simulink model "LQR_Controller_Quadrotor"  (R2019b)
settings: Solver=VariableStepAuto  StartTime=0.0  StopTime=10.0  RelTol=1e-3
values from neighbouring files (symbols this model uses):
  A = [ 0 0 0 1 0 0 0 0 0 0 0 0 ... (first row only)    [LQR control.m]
  B = [ 0 0 0 0 ... (first row only)    [LQR control.m]
  b = 6.66e-5    (= 6.66e-05)    [LQR control.m]    (also in Parameters for PID.m)
  C = [1 0 0 0 0 0 0 0 0 0 0 0 ... (first row only)    [LQR control.m]
  k = 1.642e-4    (= 0.0001642)    [LQR control.m]
  K = lqr(A,B,Q,R)    [LQR control.m]
settings Model: Creator=Dell  LastModifiedBy=Dell

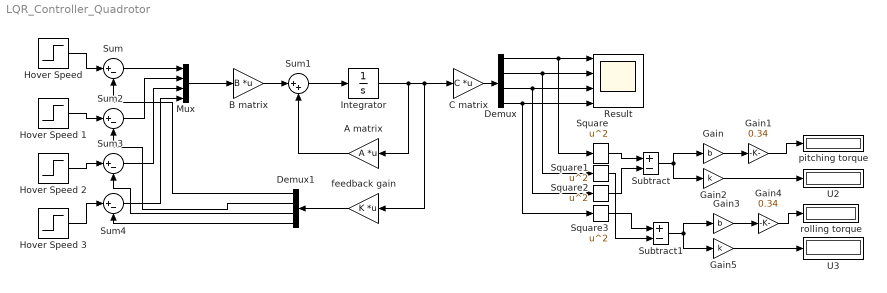
== system LQR_Controller_Quadrotor ==
  A matrix : Gain  Gain=A  Multiplication=Matrix(K*u)
  B matrix : Gain  Gain=B  Multiplication=Matrix(K*u)
  "C matrix " : Gain  Gain=C  Multiplication=Matrix(K*u)
  Demux : Demux
  Demux1 : Demux
  Gain : Gain  Gain=b
  Gain1 : Gain  Gain=0.34
  Gain2 : Gain  Gain=k
  Gain3 : Gain  Gain=b
  Gain4 : Gain  Gain=0.34
  Gain5 : Gain  Gain=k
  Hover Speed {,1..3} (4 alike) : Step  Time=1690  Before=160  SampleTime=0
  "Integrator " : Integrator  InitialCondition=1
  Mux : Mux
  Result : Scope  NumInputPorts=4
  Square{,1..3} (4 alike) : Math  Operator=square  SignedPower=off  SaturateOnIntegerOverflow=on
  Subtract : Sum  Inputs=+-
  Subtract1 : Sum  Inputs=+-
  Sum{,2..4} (4 alike) : Sum  Inputs=|+-
  Sum1 : Sum  Inputs=|++
  U2 : Display
  U3 : Display
  "feedback gain " : Gain  Gain=K  Multiplication=Matrix(K*u)
  pitching torque : Display
  rolling torque : Display
  wires:
  "C matrix "/1 -> Demux/1
  Demux/1 -> Result/1, Square/1
  Demux/2 -> Result/2, Square1/1
  Demux/3 -> Result/3, Square2/1
  Demux/4 -> Result/4, Square3/1
  Mux/1 -> B matrix/1
  B matrix/1 -> Sum1/1
  Sum1/1 -> "Integrator "/1
  "Integrator "/1 -> A matrix/1, "feedback gain "/1, "C matrix "/1
  A matrix/1 -> Sum1/2
  "Hover Speed "/1 -> Sum/1
  Sum/1 -> Mux/1
  Hover Speed 3/1 -> Sum4/1
  Hover Speed 2/1 -> Sum3/1
  Hover Speed 1/1 -> Sum2/1
  Sum2/1 -> Mux/2
  Sum3/1 -> Mux/3
  Sum4/1 -> Mux/4
  "feedback gain "/1 -> Demux1/1
  Demux1/1 -> Sum/2
  Demux1/2 -> Sum2/2
  Demux1/3 -> Sum3/2
  Demux1/4 -> Sum4/2
  Square/1 -> Subtract/1
  Square2/1 -> Subtract/2
  Square3/1 -> Subtract1/1
  Square1/1 -> Subtract1/2
  Gain/1 -> Gain1/1
  Subtract/1 -> Gain2/1, Gain/1
  Gain2/1 -> U2/1
  Gain1/1 -> pitching torque/1
  Subtract1/1 -> Gain5/1, Gain3/1
  Gain3/1 -> Gain4/1
  Gain5/1 -> U3/1
  Gain4/1 -> rolling torque/1
